simulink model "dynsim_test_urdf"  (R2020a)
settings: Solver=FixedStepAuto  StartTime=0.0  StopTime=10.0  FixedStep=0.001  RelTol=1e-3
libraries: robotmaniplib x2
settings Model: Creator=bascetta  LastModifiedBy=giuli
settings OptimizationCC: EnhancedBackFolding=on  PassReuseOutputArgsAs=Individual arguments  ZeroExternalMemoryAtStartup=off  ZeroInternalMemoryAtStartup=off  MaxStackSize=64  OptimizeBlockOrder=speed  DifferentSizesBufferReuse=on  OptimizationCustomize=off  EfficientTunableParamExpr=on
settings DebuggingCC: ParameterTunabilityLossMsg=error
settings HardwareCC: ProdBitPerPointer=32  ProdBitPerSizeT=32  ProdBitPerPtrDiffT=32  ProdLargestAtomicFloat=None  ProdIntDivRoundTo=Undefined  ProdEndianess=Unspecified  ProdWordSize=32  ProdHWDeviceType=Generic->Unspecified (assume 32-bit Generic)
settings RTWCC: SystemTargetFile=ert.tlc  HardwareBoard=Robot Operating System (ROS)  TemplateMakefile=ert_default_tmf  GenerateReport=on  Toolchain=Catkin  IncludeHyperlinkInReport=on  LaunchReport=on  TargetLang=C++  GenerateTraceInfo=on  GenerateTraceReport=on  GenerateTraceReportSl=on  GenerateTraceReportSf=on  GenerateTraceReportEml=on
settings CodeAppCC: ForceParamTrailComments=on  IgnoreCustomStorageClasses=off  OperatorAnnotations=on  SimulinkDataObjDesc=on  SFDataObjDesc=on  InsertBlockDesc=on
settings ERTTargetCC: SupportContinuousTime=on  SupportVariableSizeSignals=on

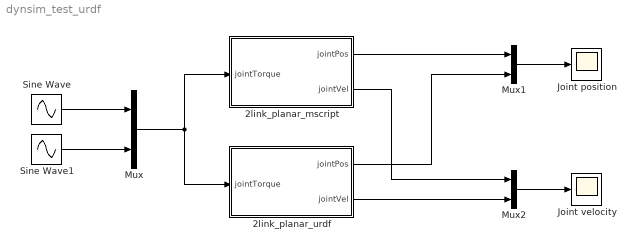
== system dynsim_test_urdf ==
  2link_planar_mscript : Subsystem
  2link_planar_urdf : Subsystem
  Joint position : Scope
  Joint velocity : Scope
  Mux : Mux  Inputs=2
  Mux1 : Mux  Inputs=2
  Mux2 : Mux  Inputs=2
  Sine Wave : Sin  Amplitude=0.01  Frequency=5  SampleTime=0
  Sine Wave1 : Sin  Amplitude=0.005  Frequency=5  SampleTime=0
  wires:
  Mux/1 -> 2link_planar_urdf/1(jointTorque), 2link_planar_mscript/1(jointTorque)
  Sine Wave1/1 -> Mux/2
  Sine Wave/1 -> Mux/1
  Mux1/1 -> Joint position/1
  2link_planar_mscript/1(jointPos) -> Mux1/1
  2link_planar_urdf/1(jointPos) -> Mux1/2
  Mux2/1 -> Joint velocity/1
  2link_planar_urdf/2(jointVel) -> Mux2/2
  2link_planar_mscript/2(jointVel) -> Mux2/1

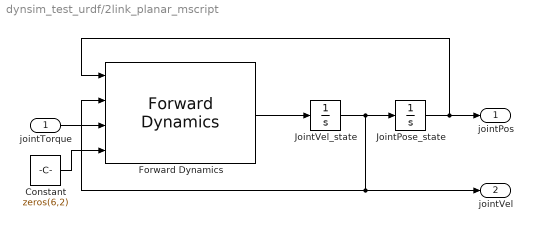
== system dynsim_test_urdf/2link_planar_mscript ==
  jointTorque : Inport
  Constant : Constant  Value=zeros(6,2)
  Forward Dynamics : robotmaniplib/Forward Dynamics  RigidBodyTree=robot_2link  SimulateUsing=Interpreted execution
  JointPose_state : Integrator  InitialCondition=[0 0]
  JointVel_state : Integrator  InitialCondition=[0 0]
  jointPos : Outport
  jointVel : Outport  Port=2
  wires:
  JointPose_state/1 -> jointPos/1, Forward Dynamics/1
  Constant/1 -> Forward Dynamics/4
  jointTorque/1 -> Forward Dynamics/3
  JointVel_state/1 -> jointVel/1, Forward Dynamics/2, JointPose_state/1
  Forward Dynamics/1 -> JointVel_state/1

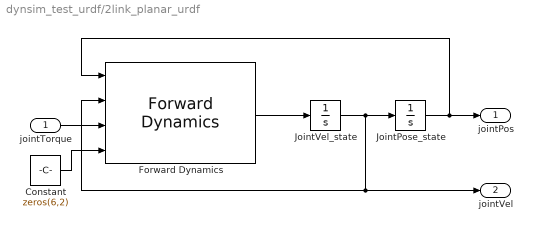
== system dynsim_test_urdf/2link_planar_urdf ==
  jointTorque : Inport
  Constant : Constant  Value=zeros(6,2)
  Forward Dynamics : robotmaniplib/Forward Dynamics  RigidBodyTree=robot_2link_fromURDF  SimulateUsing=Interpreted execution
  JointPose_state : Integrator  InitialCondition=[0 0 0]
  JointVel_state : Integrator  InitialCondition=[0 0 0]
  jointPos : Outport
  jointVel : Outport  Port=2
  wires:
  Forward Dynamics/1 -> JointVel_state/1
  JointVel_state/1 -> JointPose_state/1, Forward Dynamics/2, jointVel/1
  jointTorque/1 -> Forward Dynamics/3
  Constant/1 -> Forward Dynamics/4
  JointPose_state/1 -> Forward Dynamics/1, jointPos/1
